simulink model "update_entry_model"  (R2020b)
settings: Solver=FixedStepDiscrete  StartTime=0.0  StopTime=0.1  FixedStep=0.1  RelTol=1e-3
undefined symbols (not defined in the file or in its folder): kConsecutiveIndexDelta, kContainerLength, test_input
libraries: move_index_lib x2
settings Model: Creator=rsub  LastModifiedBy=rsub

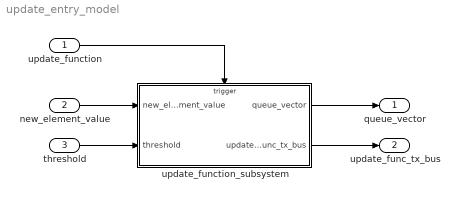
== system update_entry_model ==
  update_function : Inport  OutputFunctionCall=on
  new_element_value : Inport  Port=2  OutDataTypeStr=uint8
  threshold : Inport  Port=3  OutDataTypeStr=uint8
  update_function_subsystem : Subsystem
  queue_vector : Outport
  update_func_tx_bus : Outport  Port=2  OutDataTypeStr=Bus: update_func_tx_bus_type  BusOutputAsStruct=on
  wires:
  threshold/1 -> update_function_subsystem/2(threshold)
  new_element_value/1 -> update_function_subsystem/1(new_element_value)
  update_function/1 -> update_function_subsystem/Trigger
  update_function_subsystem/1(queue_vector) -> queue_vector/1
  update_function_subsystem/2(update_func_tx_bus) -> update_func_tx_bus/1

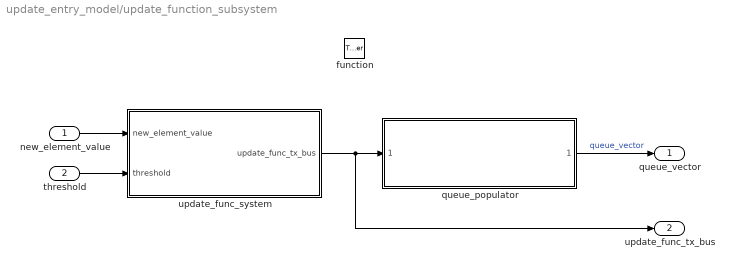
== system update_entry_model/update_function_subsystem ==
  new_element_value : Inport
  threshold : Inport  Port=2
  function : TriggerPort  TriggerType=function-call  VariantControl=Variant
  queue_populator : Subsystem  ReferencedSubsystem=queue_populator_model
  update_func_system : Subsystem
  queue_vector : Outport  SourceOfInitialOutputValue=Input signal
  update_func_tx_bus : Outport  Port=2  SourceOfInitialOutputValue=Input signal
  wires:
  new_element_value/1 -> update_func_system/1(new_element_value)
  threshold/1 -> update_func_system/2(threshold)
  queue_populator/1 -> queue_vector/1  "queue_vector"
  update_func_system/1(update_func_tx_bus) -> queue_populator/1, update_func_tx_bus/1

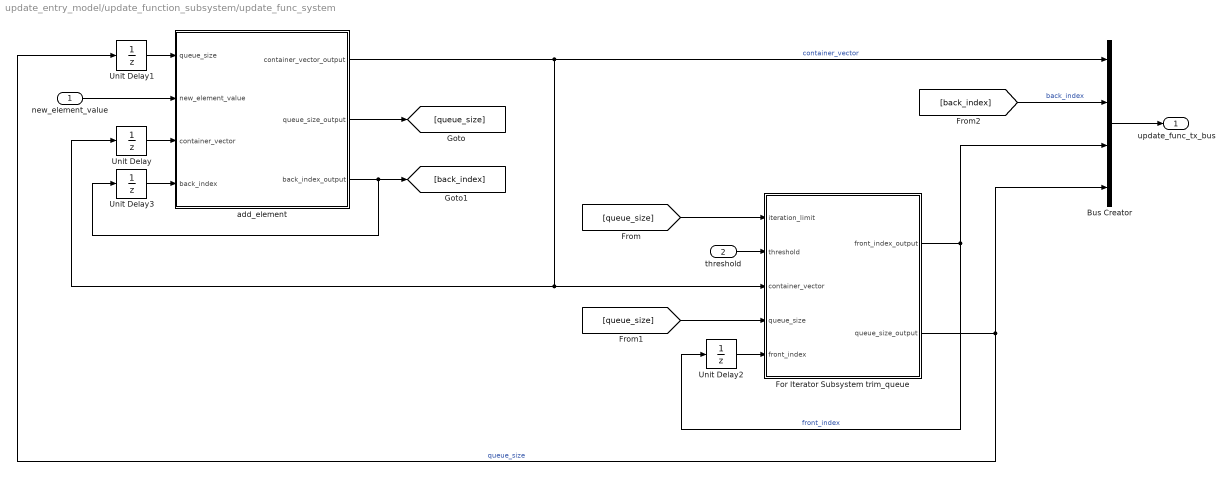
== system update_entry_model/update_function_subsystem/update_func_system ==
  new_element_value : Inport
  threshold : Inport  Port=2
  Bus Creator : BusCreator  Inputs=4  OutDataTypeStr=Bus: update_func_tx_bus_type  NonVirtualBus=on
  For Iterator Subsystem trim_queue : Subsystem  TreatAsAtomicUnit=on
  Unit Delay : UnitDelay  InitialCondition=test_input.test_container  SampleTime=-1  HasFrameUpgradeWarning=on
  Unit Delay1 : UnitDelay  InitialCondition=test_input.queue_size_starting  SampleTime=-1  HasFrameUpgradeWarning=on
  Unit Delay2 : UnitDelay  InitialCondition=test_input.front_index  SampleTime=-1  HasFrameUpgradeWarning=on
  Unit Delay3 : UnitDelay  InitialCondition=test_input.back_index_start  SampleTime=-1  HasFrameUpgradeWarning=on
  add_element : Subsystem
  update_func_tx_bus : Outport
  wires:
  new_element_value/1 -> add_element/2(new_element_value)
  threshold/1 -> For Iterator Subsystem trim_queue/2(threshold)
  For Iterator Subsystem trim_queue/2(queue_size_output) -> Bus Creator/4, Unit Delay1/1  "queue_size"
  add_element/3(back_index_output) -> [back_index], Unit Delay3/1
  add_element/1(container_vector_output) -> Bus Creator/1, Unit Delay/1, For Iterator Subsystem trim_queue/3(container_vector)  "container_vector"
  Unit Delay2/1 -> For Iterator Subsystem trim_queue/5(front_index)
  [queue_size] -> For Iterator Subsystem trim_queue/1(iteration_limit)
  Unit Delay1/1 -> add_element/1(queue_size)
  Unit Delay/1 -> add_element/3(container_vector)
  Unit Delay3/1 -> add_element/4(back_index)
  add_element/2(queue_size_output) -> [queue_size]
  For Iterator Subsystem trim_queue/1(front_index_output) -> Bus Creator/3, Unit Delay2/1  "front_index"
  [queue_size] -> For Iterator Subsystem trim_queue/4(queue_size)
  Bus Creator/1 -> update_func_tx_bus/1
  [back_index] -> Bus Creator/2  "back_index"

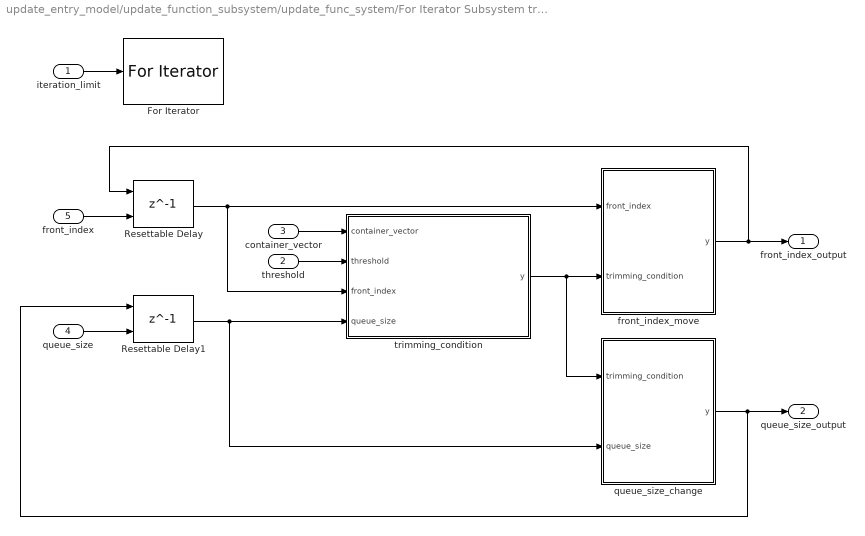
== system update_entry_model/update_function_subsystem/update_func_system/For Iterator Subsystem trim_queue ==
  iteration_limit : Inport
  threshold : Inport  Port=2
  container_vector : Inport  Port=3
  queue_size : Inport  Port=4
  front_index : Inport  Port=5
  For Iterator : ForIterator  ResetStates=reset  IterationSource=external  IterationLimit=kContainerLength  ShowIterationPort=off  IndexMode=Zero-based  IterationVariableDataType=uint8
  Resettable Delay : Delay  DelayLength=1  InitialConditionSource=Input port
      settings: InputPortMap=u0,p4
  Resettable Delay1 : Delay  DelayLength=1  InitialConditionSource=Input port
      settings: InputPortMap=u0,p4
  front_index_move : Subsystem
  queue_size_change : Subsystem
  trimming_condition : Subsystem
  front_index_output : Outport  InitialOutput=test_input.front_index
  queue_size_output : Outport  Port=2  InitialOutput=test_input.queue_size_starting
  wires:
  queue_size/1 -> Resettable Delay1/2
  front_index/1 -> Resettable Delay/2
  Resettable Delay/1 -> trimming_condition/3(front_index), front_index_move/1(front_index)
  Resettable Delay1/1 -> trimming_condition/4(queue_size), queue_size_change/2(queue_size)
  iteration_limit/1 -> For Iterator/1
  trimming_condition/1(y) -> queue_size_change/1(trimming_condition), front_index_move/2(trimming_condition)
  container_vector/1 -> trimming_condition/1(container_vector)
  threshold/1 -> trimming_condition/2(threshold)
  queue_size_change/1(y) -> queue_size_output/1, Resettable Delay1/1
  front_index_move/1(y) -> front_index_output/1, Resettable Delay/1

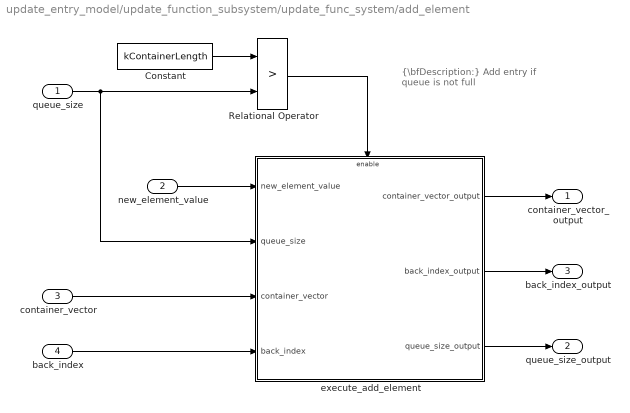
== system update_entry_model/update_function_subsystem/update_func_system/add_element ==
  note: {\bfDescription:}
      | Add entry if queue is not full
  queue_size : Inport
  new_element_value : Inport  Port=2
  container_vector : Inport  Port=3
  back_index : Inport  Port=4
  Constant : Constant  Value=kContainerLength
  Relational Operator : RelationalOperator  Operator=>  OutDataTypeStr=boolean  RndMeth=Simplest
  execute_add_element : Subsystem
  container_vector_output : Outport
  queue_size_output : Outport  Port=2
  back_index_output : Outport  Port=3
  wires:
  execute_add_element/3(queue_size_output) -> queue_size_output/1
  Relational Operator/1 -> execute_add_element/Enable
  new_element_value/1 -> execute_add_element/1(new_element_value)
  execute_add_element/2(back_index_output) -> back_index_output/1
  execute_add_element/1(container_vector_output) -> container_vector_output/1
  container_vector/1 -> execute_add_element/3(container_vector)
  back_index/1 -> execute_add_element/4(back_index)
  Constant/1 -> Relational Operator/1
  queue_size/1 -> Relational Operator/2, execute_add_element/2(queue_size)

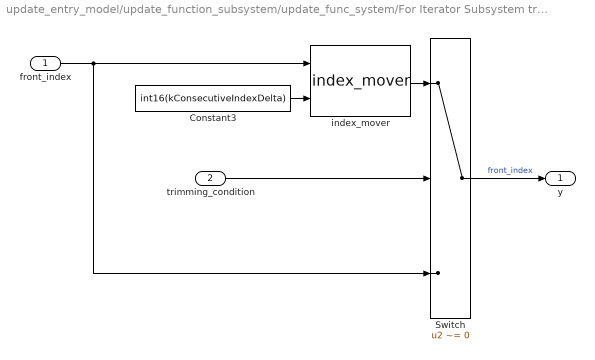
== system update_entry_model/update_function_subsystem/update_func_system/For Iterator Subsystem trim_queue/front_index_move ==
  front_index : Inport
  trimming_condition : Inport  Port=2
  Constant3 : Constant  Value=int16(kConsecutiveIndexDelta)
  Switch : Switch  Criteria=u2 ~= 0
  index_mover : move_index_lib/index_mover  SystemSampleTime=-1  VariantActivationTime=update diagram  Latency=0  AutoFrameSizeCalculation=off
  y : Outport
  wires:
  front_index/1 -> Switch/3, index_mover/1
  index_mover/1 -> Switch/1
  Switch/1 -> y/1  "front_index"
  trimming_condition/1 -> Switch/2
  Constant3/1 -> index_mover/2

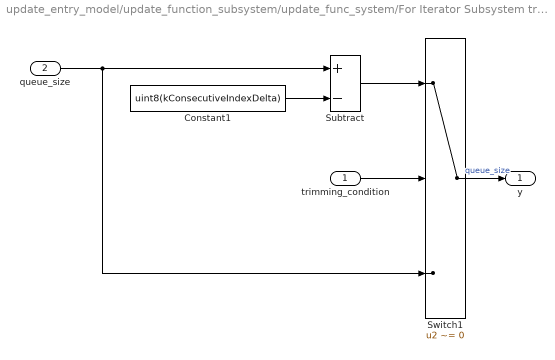
== system update_entry_model/update_function_subsystem/update_func_system/For Iterator Subsystem trim_queue/queue_size_change ==
  trimming_condition : Inport
  queue_size : Inport  Port=2
  Constant1 : Constant  Value=uint8(kConsecutiveIndexDelta)
  Subtract : Sum  Inputs=+-
  Switch1 : Switch  Criteria=u2 ~= 0
  y : Outport
  wires:
  Switch1/1 -> y/1  "queue_size"
  trimming_condition/1 -> Switch1/2
  Subtract/1 -> Switch1/1
  queue_size/1 -> Switch1/3, Subtract/1
  Constant1/1 -> Subtract/2

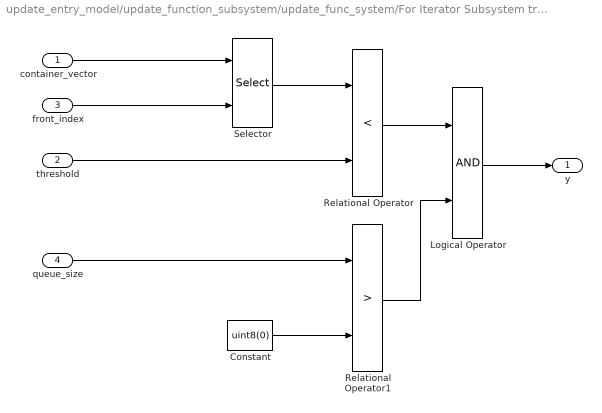
== system update_entry_model/update_function_subsystem/update_func_system/For Iterator Subsystem trim_queue/trimming_condition ==
  container_vector : Inport
  threshold : Inport  Port=2
  front_index : Inport  Port=3
  queue_size : Inport  Port=4
  Constant : Constant  Value=uint8(0)
  Logical Operator : Logic  AllPortsSameDT=off  OutDataTypeStr=boolean
  Relational Operator : RelationalOperator  Operator=<  OutDataTypeStr=boolean  RndMeth=Simplest
  Relational Operator1 : RelationalOperator  Operator=>  OutDataTypeStr=boolean  RndMeth=Simplest
  Selector : Selector  IndexMode=Zero-based  InputPortWidth=kContainerLength  IndexOptions=Index vector (port)  Indices=[1 3]  OutputSizes=1
  y : Outport
  wires:
  container_vector/1 -> Selector/1
  queue_size/1 -> Relational Operator1/1
  Logical Operator/1 -> y/1
  Selector/1 -> Relational Operator/1
  Relational Operator1/1 -> Logical Operator/2
  threshold/1 -> Relational Operator/2
  front_index/1 -> Selector/2
  Relational Operator/1 -> Logical Operator/1
  Constant/1 -> Relational Operator1/2

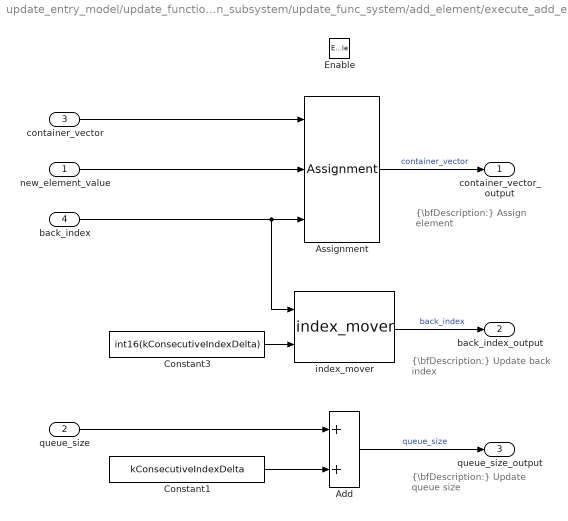
== system update_entry_model/update_function_subsystem/update_func_system/add_element/execute_add_element ==
  note: {\bfDescription:}
      | Update queue size
  note: {\bfDescription:}
      | Update back index
  note: {\bfDescription:}
      | Assign element
  new_element_value : Inport
  queue_size : Inport  Port=2
  container_vector : Inport  Port=3
  back_index : Inport  Port=4
  Enable : EnablePort  StatesWhenEnabling=reset
  Add : Sum
  Assignment : Assignment  IndexMode=Zero-based  DiagnosticForDimensions=Warning  IndexOptions=Index vector (port)  Indices=1  OutputSizes=1
  Constant1 : Constant  Value=kConsecutiveIndexDelta
  Constant3 : Constant  Value=int16(kConsecutiveIndexDelta)
  index_mover : move_index_lib/index_mover  SystemSampleTime=-1  VariantActivationTime=update diagram  Latency=0  AutoFrameSizeCalculation=off
  container_vector_output : Outport  InitialOutput=test_input.test_container
  back_index_output : Outport  Port=2  InitialOutput=test_input.back_index_start
  queue_size_output : Outport  Port=3  InitialOutput=test_input.queue_size_starting
  wires:
  index_mover/1 -> back_index_output/1  "back_index"
  Add/1 -> queue_size_output/1  "queue_size"
  Assignment/1 -> container_vector_output/1  "container_vector"
  back_index/1 -> index_mover/1, Assignment/3
  Constant1/1 -> Add/2
  queue_size/1 -> Add/1
  Constant3/1 -> index_mover/2
  container_vector/1 -> Assignment/1
  new_element_value/1 -> Assignment/2
